simulink model "positionctrl_virt"  (Simulink 6.6)
settings: Solver=ode45  StartTime=0.0  StopTime=3  RelTol=1e-3
StopFcn:
  | save_system(vars.simfilename);
libraries: simulink_extras x1
CloseFcn:
  | save_system(vars.simfilename); sim(vars.simfilename);vars.simtime = str2num(get_param(vars.simfilename,'StopTime'));set(guiel.hSimtime,'String',num2str(vars.simtime));if strcmp(vars.simfilename(end-2:end),'sim') vars.L= motorParams(1,1); vars.R= motorParams(1,2); vars.J= motorParams(1,3);vars.b= motorParams(1,4); vars.Kb= motorParams(1,5); vars.Km= motorParams(1,6);if (min(size(motorParams)) == 9) vars.P= motorParams(1,7); vars.I= motorParams(1,8); vars.D= motorParams(1,9);else;vars.P= NaN; vars.I= NaN; vars.D= NaN;end;clear motorParams; [vars.numericTF vars.symbolTF] = calcTF2(vars);end,
settings Model: Creator=Farid Golnaraghi  LastModifiedBy=Farid Golnaraghi
settings DataIOCC: MaxDataPoints=10000
settings OptimizationCC: BlockReduction=off  BooleanDataType=off
settings DebuggingCC: SignalResolutionControl=TryResolveAllWithWarning  SolverPrmCheckMsg=none  MultiTaskDSMMsg=warning  MultiTaskCondExecSysMsg=none  StrictBusMsg=None
settings HardwareCC: TargetUnknown=on
settings RTWCC: IncludeERTFirstTime=on

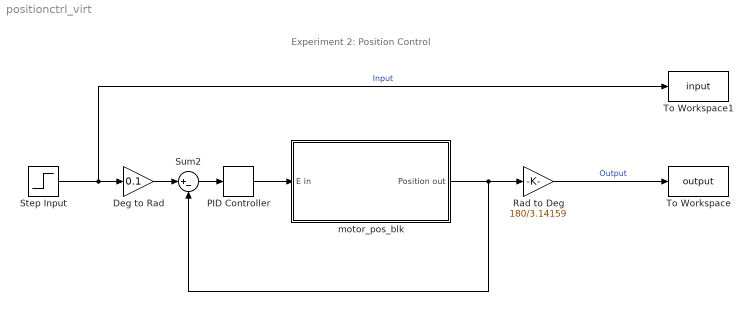
== system positionctrl_virt ==
  note: Experiment 2: Position Control
  Deg to Rad : Gain  Gain=0.1  SaturateOnIntegerOverflow=on
  PID Controller : simulink_extras/Additional Linear/PID Controller  SystemSampleTime=-1  P=1  I=0  D=0.1
  Rad to Deg : Gain  Gain=180/3.14159  SaturateOnIntegerOverflow=on
  Step Input : Step  Time=0  SampleTime=0
  Sum2 : Sum  Inputs=|+-  SaturateOnIntegerOverflow=on  InputSameDT=on
  To Workspace : ToWorkspace  VariableName=output  SampleTime=-1  SaveFormat=Structure With Time
  To Workspace1 : ToWorkspace  VariableName=input  SampleTime=-1  SaveFormat=Structure With Time
  motor_pos_blk : Subsystem
      mask Description: Real-Time Workshop generated S-function.
      mask Help: web(['file://',docroot,'/toolbox/rtw/rtwsfcn.html']);
      mask Display: disp('DC Motor (Position Control)')
  wires:
  Rad to Deg/1 -> To Workspace/1  "Output"
  motor_pos_blk/1(Position out) -> Sum2/2, Rad to Deg/1
  PID Controller/1 -> motor_pos_blk/1(E in)
  Sum2/1 -> PID Controller/1
  Deg to Rad/1 -> Sum2/1
  Step Input/1 -> Deg to Rad/1, To Workspace1/1  "Input"

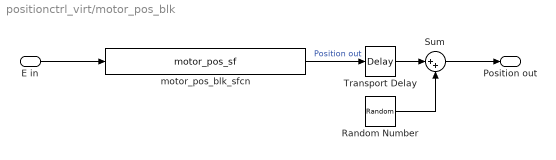
== system positionctrl_virt/motor_pos_blk ==
  E in : Inport
  Random Number : RandomNumber  Variance=0.000005  SampleTime=0.005
  Sum : Sum  Inputs=|++  SaturateOnIntegerOverflow=on  InputSameDT=on
  Transport Delay : TransportDelay  DelayTime=0.001  BufferSize=10000
  motor_pos_blk_sfcn : S-Function  FunctionName=motor_pos_sf  SFunctionModules=""  mask{rtw_sf_name=motor_pos_sf, showVar=off}
      mask prompts: rtw_sf_name "Generated S-function name (model_sf):"; showVar "Show module list"
      mask help: Real-Time Workshop generated S-function.
      mask init:
      | displist = '';
      | if ~strcmp(get_param(gcb, 'FunctionName'), rtw_sf_name);
      |   set_param(gcb, 'FunctionName', rtw_sf_name);
      | end
      | if  showVar & exist('rtwsfunc') == 2
      |   tmplist = rtwsfunc(rtw_sf_name,gcb);
      |   tmplist = ['\nList of Modules:\n', tmplist];
      | elseif showVar
      |   tmplist = '\nList of Modules:\nRTW not licensed\n';
      | end
      | if showVar
      |   displist = tmplist;
      | end
      settings: CopyFcn=set_param(gcb,'linkstatus','none')
      mask Help: web(['file://',docroot,'/toolbox/rtw/rtwsfcn.html']);
      mask Display:
      | port_label('input',1,'E in');
      | port_label('output',1,'Position out');
  Position out : Outport
  wires:
  Random Number/1 -> Sum/2
  Sum/1 -> Position out/1
  Transport Delay/1 -> Sum/1
  motor_pos_blk_sfcn/1 -> Transport Delay/1  "Position out"
  E in/1 -> motor_pos_blk_sfcn/1
